simulink model "my_DC_motor_control_position"  (R2022b)
settings: Solver=VariableStepAuto  StartTime=0.0  StopTime=10  FixedStep=0.0001  RelTol=1e-3
values from neighbouring files (symbols this model uses):
  B_motor = 1.9099e-4    (= 0.00019099)    [DC_motor_init.m]    (also in LOAD_ROBOT_DATA.m = 0.000678; circular_interp.m = 0.000678; computed_torque_control.m; create_model_tree.m)
  J_rotor = 2118.45e-7    (= 0.000211845)    [DC_motor_init.m]    (also in LOAD_ROBOT_DATA.m = 0.0125; circular_interp.m = 0.0125; computed_torque_control.m; create_model_tree.m)
  Ke = 0.08    [DC_motor_init.m]    (also in LOAD_ROBOT_DATA.m = 0.957; circular_interp.m = 0.957; computed_torque_control.m; create_model_tree.m)
  Kt = 0.08    [DC_motor_init.m]    (also in LOAD_ROBOT_DATA.m = 0.957; circular_interp.m = 0.957; computed_torque_control.m; create_model_tree.m)
  L = 0.90e-3    (= 0.0009)    [DC_motor_init.m]    (also in LOAD_ROBOT_DATA.m = 0.0054; circular_interp.m = 0.0054; computed_torque_control.m; create_model_tree.m)
  lower_sat_voltage = 0    [DC_motor_init.m]    (also in LOAD_ROBOT_DATA.m; circular_interp.m; computed_torque_control.m; create_model_tree.m)
  R = 0.43    [DC_motor_init.m]    (also in LOAD_ROBOT_DATA.m = 1.45; circular_interp.m = 1.45; computed_torque_control.m; create_model_tree.m)
  T_disturbance = 1    [DC_motor_init.m]
  upper_sat_voltage = 30    [DC_motor_init.m]    (also in LOAD_ROBOT_DATA.m; circular_interp.m; computed_torque_control.m; create_model_tree.m)
libraries: slpidlib x1
settings Model: Creator=doann  LastModifiedBy=doann

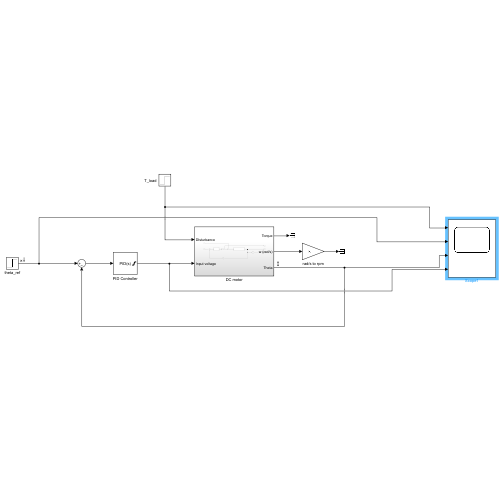
[thumbnail: Simulink's stored preview of the top-level diagram]
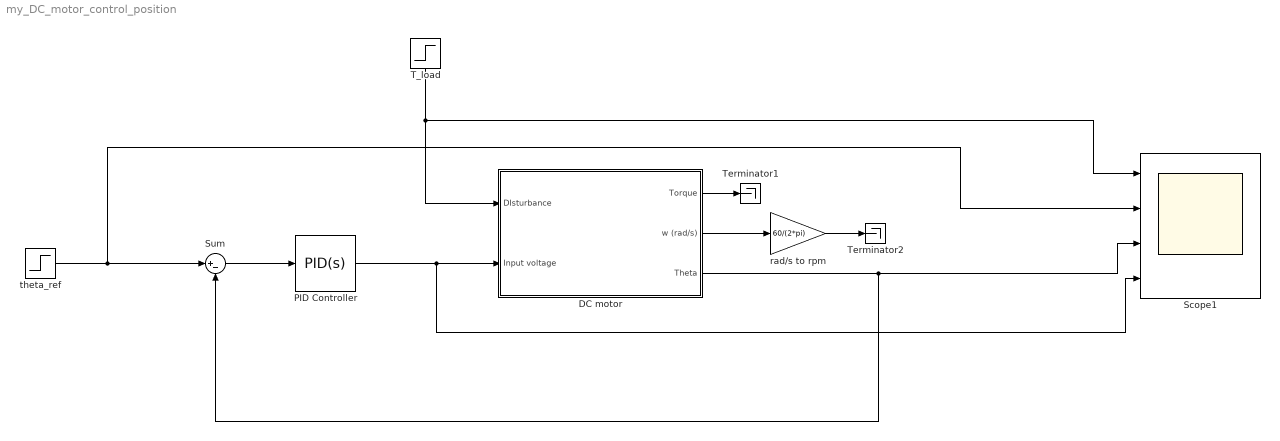
== system my_DC_motor_control_position ==
  DC motor : Subsystem
  PID Controller : slpidlib/PID Controller  Controller=PID  Form=Parallel  TimeDomain=Continuous-time  UseExternalTs=off  SampleTime=-1  IntegratorMethod=Forward Euler  FilterMethod=Forward Euler  ControllerParametersSource=internal  P=6.64964216151724  I=8.47711277932516  UseKiTs=off  D=0.168344697084415  N=17225.0588911599  UseFilter=on  TunerSelectOption=Transfer Function Based (PID Tuner App)  InitialConditionSource=internal  InitialConditionForIntegrator=lower_sat_voltage  InitialConditionForFilter=lower_sat_voltage  DifferentiatorICPrevScaledInput=0  ExternalReset=none  TrackingMode=off  Kt=1  LimitOutput=on  SatLimitsSource=internal  UpperSaturationLimit=upper_sat_voltage  LowerSaturationLimit=lower_sat_voltage  LinearizeAsGain=on  AntiWindupMode=none  Kb=1  LimitIntegrator=off  UpperIntegratorSaturationLimit=inf  LowerIntegratorSaturationLimit=-inf  POutMin=[]  POutMax=[]  IOutMin=[]  IOutMax=[]  DOutMin=[]  DOutMax=[]  NOutMin=[]  NOutMax=[]  SumOutMin=[]  SumOutMax=[]  SaturationOutMin=[]  SaturationOutMax=[]  PParamMin=[]  PParamMax=[]  IParamMin=[]  IParamMax=[]  DParamMin=[]  DParamMax=[]  NParamMin=[]  NParamMax=[]  KbParamMin=[]  KbParamMax=[]  KtParamMin=[]  KtParamMax=[]  KbOutMin=[]  KbOutMax=[]  KtOutMin=[]  KtOutMax=[]  IntegratorOutMin=[]  IntegratorOutMax=[]  FilterOutMin=[]  FilterOutMax=[]  SumI1OutMin=[]  SumI1OutMax=[]  SumI2OutMin=[]  SumI2OutMax=[]  SumI3OutMin=[]  SumI3OutMax=[]  SumI4OutMin=[]  SumI4OutMax=[]  SumDOutMin=[]  SumDOutMax=[]  DifferentiatorOutMin=[]  DifferentiatorOutMax=[]  FilterDiffOutCoefMin=[]  FilterDiffOutCoefMax=[]  ReciprocalOutMin=[]  ReciprocalOutMax=[]  SumDenOutMin=[]  SumDenOutMax=[]  SumNumOutMin=[]  SumNumOutMax=[]  DivideOutMin=[]  DivideOutMax=[]  UdiffTsProdOutMin=[]  UdiffTsProdOutMax=[]  NTsProdOutMin=[]  NTsProdOutMax=[]  UintegralTsProdOutMin=[]  UintegralTsProdOutMax=[]  UngainTsProdOutMin=[]  UngainTsProdOutMax=[]  ClampingZeroOutDataTypeStr=Inherit: Inherit via back propagation  ClampingZeroOutMin=[]  ClampingZeroOutMax=[]  FilterDenConstantOutDataTypeStr=Inherit: Inherit via back propagation  FilterDenConstantOutMin=[]  FilterDenConstantOutMax=[]  PCopyOutDataTypeStr=Inherit: Inherit via back propagation  PCopyOutMin=[]  PCopyOutMax=[]  NCopyOutDataTypeStr=Inherit: Inherit via back propagation  NCopyOutMin=[]  NCopyOutMax=[]  IntegratorContinuousStateAttributes=''  IntegratorStateMustResolveToSignalObject=off  IntegratorRTWStateStorageClass=Auto  FilterContinuousStateAttributes=''  FilterStateMustResolveToSignalObject=off  FilterRTWStateStorageClass=Auto  ParallelPVariant=InternalParameters  IdealPVariant=Disabled  IVariant=InternalParameters  DVariant=InternalParameters  IntegratorVariant=Continuous  SatVariant=Enabled  AWVariant=Passthrough  PCopyVariant=Disabled  TRVariant=Disabled  FdbkBlocksVariant=Forward  IdealPFdbkVariant=Disabled  SatFdbkVariant=Disabled  DerivativeFilterVariant=ContFilter  NVariant=InternalParameters  NCopyVariant=Disabled  FilterICVariant=InternalICsFilter  IntegratorICVariant=InternalICs  ExternalResetVariant=Disabled  TRSumVariant=Passthrough  SumFdbkVariant=Disabled  SumVariant=Sum_PID  TsampFilterVariant=InternalTs  TsampNgainVariant=Passthrough  TsampIntegralVariant=Passthrough  ExternalSaturationOutDataTypeStr=Inherit: Same as second input
  Scope1 : Scope  NumInputPorts=4
  Sum : Sum  Inputs=|+-
  T_load : Step  Time=2.5  After=T_disturbance  SampleTime=0
  Terminator1 : Terminator
  Terminator2 : Terminator
  rad/s to rpm : Gain  Gain=60/(2*pi)
  theta_ref : Step  After=pi  SampleTime=0
  wires:
  rad/s to rpm/1 -> Terminator2/1
  PID Controller/1 -> Scope1/4, DC motor/2(Input voltage)
  T_load/1 -> Scope1/1, DC motor/1(DIsturbance)
  DC motor/2(w (rad/s)) -> rad/s to rpm/1
  DC motor/1(Torque) -> Terminator1/1
  DC motor/3(Theta) -> Scope1/3, Sum/2
  theta_ref/1 -> Sum/1, Scope1/2
  Sum/1 -> PID Controller/1

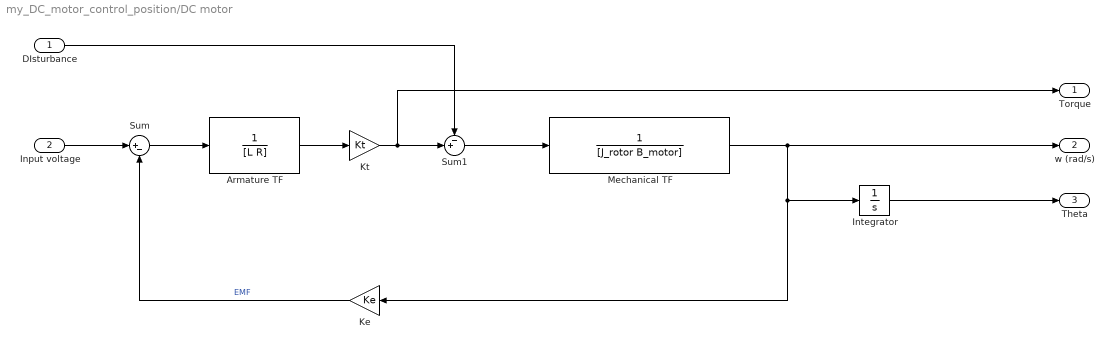
== system my_DC_motor_control_position/DC motor ==
  DIsturbance : Inport
  Input voltage : Inport  Port=2
  Armature TF : TransferFcn  Denominator=[L R]
  Integrator : Integrator
  Ke : Gain  Gain=Ke
  Kt : Gain  Gain=Kt
  Mechanical TF : TransferFcn  Denominator=[J_rotor B_motor]
  Sum : Sum  Inputs=|+-
  Sum1 : Sum  Inputs=-+|
  Torque : Outport
  w (rad/s) : Outport  Port=2
  Theta : Outport  Port=3
  wires:
  Ke/1 -> Sum/2  "EMF"
  Mechanical TF/1 -> w (rad/s)/1, Ke/1, Integrator/1
  Kt/1 -> Torque/1, Sum1/2
  Sum/1 -> Armature TF/1
  Sum1/1 -> Mechanical TF/1
  Armature TF/1 -> Kt/1
  DIsturbance/1 -> Sum1/1
  Integrator/1 -> Theta/1
  Input voltage/1 -> Sum/1
